simulink model "GraphicalFunction2"  (R2020b)
settings: Solver=VariableStepAuto  StartTime=0.0  StopTime=0.1  RelTol=1e-3
settings Model: Creator=86188  LastModifiedBy=apple
settings DataIOCC: ReturnWorkspaceOutputs=off
settings DebuggingCC: ArithmeticOperatorsInVariantConditions=warning
settings SFSimCC: SimUseLocalCustomCode=off  CustomCodeUndefinedFunction=UseInterfaceOnly
settings RTWCC: RTWUseLocalCustomCode=off

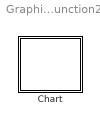
== system GraphicalFunction2 ==
  Chart : Stateflow chart  TreatAsAtomicUnit=on

== stateflow chart GraphicalFunction2/Chart ==
  state i=set(sn) [function]
    (junction 10) -> (junction 4) : {i = i + 1;f("set")}
    (junction 3) -> (junction 10) [order 1] : [i<=sn]
    (junction 4) -> (junction 3)
    (default) -> (junction 3) : {i=1;}
    (junction 3) -> (junction 9) [order 2]
  state A
    en: f("en_A");
    data=set(3);
  state B
    en: f("en_B");
  (default) -> A
  A -> B
  data: sn function_input; i function_output; s function_input; data local
  function f(s):
    | function f(s)
    |   fprintf(s+"\n");
